simulink library "speedgoatlib_fpga_analog_io"  (R2024b)
settings: Solver=VariableStepAuto  StartTime=0.0  StopTime=10.0  RelTol=1e-3
undefined symbols (not defined in the file): IO336, sg_fpga_callBackInit_m_a1, sg_fpga_io324_analog_input_m, sg_fpga_io324_analog_output_m, sg_fpga_io324_analog_setup_m, sg_fpga_io325_analog_input_m, sg_fpga_io325_analog_output_m, sg_fpga_io325_analog_setup_m, sg_fpga_io334_analog_input_m, sg_fpga_io334_analog_output_m, sg_fpga_io334_analog_setup_m, sg_fpga_io336_analog_input_m, sg_fpga_io336_analog_output_m, sg_fpga_io336_analog_setup_m, sg_fpga_io337_analog_input_m, sg_fpga_io337_analog_output_m, sg_fpga_io337_analog_setup_m, sg_fpga_io3xx_120_analog_input_m, sg_fpga_io3xx_120_analog_output_m, sg_fpga_io3xx_120_analog_setup_m
(part 1 of 4)
settings Model: Creator=Speedgoat GmbH  LastModifiedBy=speedgoat\jenkins
settings DebuggingCC: UnderspecifiedInitializationDetection=Classic  MergeDetectMultiDrivingBlocksExec=none
settings ModelReferenceCC: PropagateSignalLabelsOutOfModel=off
settings ConfigComp: CovBoundaryAbsTol=1.0e-5

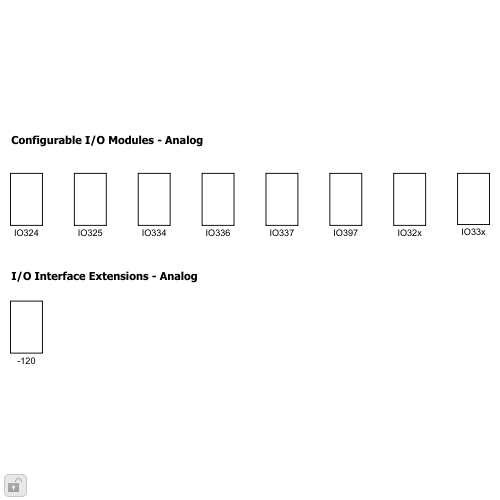
[thumbnail: Simulink's stored preview of the top-level diagram]
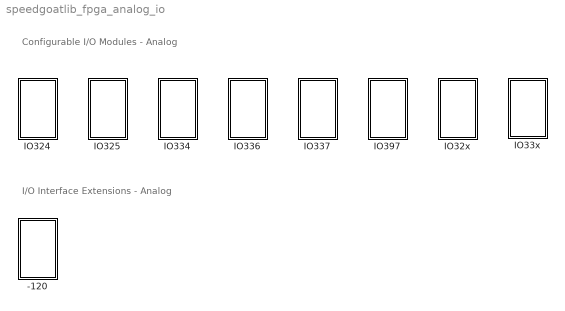
== system speedgoatlib_fpga_analog_io ==
  note: Configurable I/O Modules - Analog
  note: I/O Interface Extensions - Analog
  -120 : Subsystem
  IO324 : Subsystem
  IO325 : Subsystem
  IO32x : Subsystem
  IO334 : Subsystem
  IO336 : Subsystem
  IO337 : Subsystem
  IO33x : Subsystem
  IO397 : Subsystem

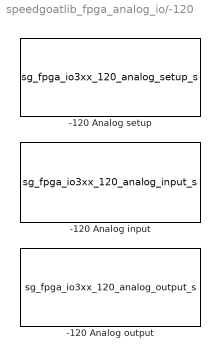
== system speedgoatlib_fpga_analog_io/-120 ==
  -120 Analog input : S-Function  InitFcn=sg_fpga_io3xx_120_analog_input_m.runInitFcn();  FunctionName=sg_fpga_io3xx_120_analog_input_s  Parameters=id, parSampleTime, parAiChannels, parAiChannelsStreamed, parAiEnableFrame, parAiFrameSize  SFunctionDeploymentMode=off  EnableBusSupport=off  mask(ad_fpga_io3xx_120){id=1, parSampleTime=-1, pciSlot=[-1,-1], parAiChannels=[1 2], parAiChannelsStreamed=[1 2], parAiTriggerMode=[2 2], parAiReadPrevValue=0, parAiEnableFrame=0, parAdcCoupling=[1 1 1 1], parAdcContSampling=0, parAdcDmaEnable=0, parAdcActiveDmaDevices=[1 1 1 1], parAiFrameSize=100}
      mask prompts: id "Configurable I/O Module ID"; parSampleTime "Sample Time [s]"
      mask help: Speedgoat Driver Block<br>Configurable I/O - 120 Analog Input<br><br>&copy; 2007 - 2026, Speedgoat GmbH, <a href="matlab: web('www.speedgoat.com','-browser');">www.speedgoat.com</a>
      mask init:
      | sg_fpga_io3xx_120_analog_input_m.runMaskInit();
      mask Help: eval('sg.utils.help.show(''io_main/refentry_120_analog_input_v1'');')
      mask TypeOptions id: 1 | 2 | 3 | 4 | 5 | 6 | 7 | 8 | 9 | 10
      mask Display: disp('Speedgoat\nConfigurable I/O\n-120 Analog input v1\nModule ID: 1');port_label('output',1,'1');port_label('output',2,'2');
  -120 Analog output : S-Function  InitFcn=sg_fpga_io3xx_120_analog_output_m.runInitFcn();  FunctionName=sg_fpga_io3xx_120_analog_output_s  Parameters=id, parSampleTime, parAoChannels, parAoEnableFrame, parAoFrameSize  SFunctionDeploymentMode=off  EnableBusSupport=off  mask(da_fpga_io3xx_120){id=1, parSampleTime=-1, pciSlot=[-1,-1], board=IO336-325k, parAoChannels=[1 2], parAoVoltageRange=[1 1], parDacOverRange=[0 0 0 0 0 0 0 0], parAoInitValues=[0 0], parAoReset=[1 1], parDacSyncOut=1, parAoEnableFrame=0, parDacActiveDmaDevices=[1 1 1 1], parDacDmaLatency=2, parAoFrameSize=1000}
      mask prompts: id "Configurable I/O Module ID"; parSampleTime "Sample Time [s]"
      mask help: Speedgoat Driver Block<br>Configurable I/O - 120 Analog Output<br><br>&copy; 2007 - 2026, Speedgoat GmbH, <a href="matlab: web('www.speedgoat.com','-browser');">www.speedgoat.com</a>
      mask init:
      | sg_fpga_io3xx_120_analog_output_m.runMaskInit();
      mask Help: eval('sg.utils.help.show(''io_main/refentry_120_analog_output_v1'');')
      mask TypeOptions id: 1 | 2 | 3 | 4 | 5 | 6 | 7 | 8 | 9 | 10
      mask Display: disp('Speedgoat\nConfigurable I/O\n-120 Analog output v1\nModule ID: 1');port_label('input',1,'1');port_label('input',2,'2');
  -120 Analog setup : S-Function  InitFcn=sg_fpga_io3xx_120_analog_setup_m.runInitFcn();  FunctionName=sg_fpga_io3xx_120_analog_setup_s  Parameters=id, p.cmcEnable, p.AdcActiveChannels, p.AdcReadPrevValue, p.AdcFilterWidthPow2, p.AdcOversamplRate, parAdcAutoCorrection, p.AdcTriggerMode, p.AdcClockDivider, p.AdcInternalTrigger, p.AdcExternalTrigger, p.AdcEnableFrame, p.AdcFrameSize, p.DacChannels, p.DacVoltageRange, p.DacInitValues, p.DacReset, parDacAutoCorrection, p.DacTriggerMode, p.DacClockDivider, p.DacInternalTrigger, p.DacExternalTrigger, p.DacEnableFrame, p.DacFifoThreshold, p.DacSourceSelection, p.DacFrameSize, p.EnableTriggerForCm, p.DacUsesTimer  SFunctionModules=sg_fpga_analog_dma sg_AnalogInputCm_IO336 sg_AnalogOutputCm_IO334  SFunctionDeploymentMode=off  EnableBusSupport=off  mask(analog_setup_fpga_io3xx_120){id=1, siteIdx=1, parEnableCodeModule1=off, parEnableCodeModule2=off, parEnableCodeModule3=off, parEnableCodeModule4=off, parEnableCodeModule5=off, parEnableCodeModule6=off, parEnableCodeModule7=off, parEnableCodeModule8=off, parAdcEnableIndividualTrigger=off, parAdcTriggerMode1=Model Step, parAdcSampleRate1=1e5, parAdcDioTriggerChannel1=1, parAdcInternalTrigger1=<empty>, parAdcOversampling1=None, parAdcTriggerMode2=Model Step, parAdcSampleRate2=1e5, parAdcDioTriggerChannel2=1, parAdcInternalTrigger2=<empty>, parAdcOversampling2=None, parAdcTriggerMode3=Model Step, parAdcSampleRate3=1e5, parAdcDioTriggerChannel3=1, parAdcInternalTrigger3=<empty>, parAdcOversampling3=None, parAdcTriggerMode4=Model Step, parAdcSampleRate4=1e5, parAdcDioTriggerChannel4=1, parAdcInternalTrigger4=<empty>, parAdcOversampling4=None, parAdcReadPrevValueIndividualTrigger=off, parAdcEnableFrame=off, parAdcTriggerMode=I/O Module Clock, parAdcReadPrevValue=on, parAdcSampleRate=100e3, parAdcDioTriggerChannel=1, parAdcInternalTrigger=<empty>, parAdcOversampling=None, parAdcTriggerResolution=1e-08, parAdcSampleRateFrame=1e5, parAdcFrameSize=100, parAdcSampleTime=-1, parDacTriggerMode=Model Step, parDacInternalTrigger=<empty>, parDacDioTriggerChannel=1, parDacEnableFrame=on, dacUsesTimer=off, parDacFifoThreshold=100, parDacTriggerResolution=1e-08, parDacSampleRate=1e6, parDacFrameSize=1000, parDacSampleTime=-1, parAdcChannel1=on, parAdcChannel2=on, parAdcChannel3=off, parAdcChannel4=off, parAdcChannel5=off, parAdcChannel6=off, parAdcChannel7=off, parAdcChannel8=off, parAdcChannel9=off, parAdcChannel10=off, parAdcChannel11=off, parAdcChannel12=off, parAdcChannel13=off, parAdcChannel14=off, parAdcChannel15=off, parAdcChannel16=off, parAdcChannel17=off, parAdcChannel18=off, parAdcChannel19=off, parAdcChannel20=off, parAdcChannel21=off, parAdcChannel22=off, parAdcChannel23=off, parAdcChannel24=off, parAdcChannel25=off, parAdcChannel26=off, parAdcChannel27=off, parAdcChannel28=off, parAdcChannel29=off, parAdcChannel30=off, parAdcChannel31=off, parAdcChannel32=off, parAdcAutoCorrection=on, parDacChannel1=on, parDacChannel2=on, parDacChannel3=off, parDacChannel4=off, parDacChannel5=off, parDacChannel6=off, parDacChannel7=off, parDacChannel8=off, parDacChannel9=off, parDacChannel10=off, parDacChannel11=off, parDacChannel12=off, parDacChannel13=off, parDacChannel14=off, parDacChannel15=off, parDacChannel16=off, parDacRange1=+-10 V, parDacInitValue1=0, parDacReset1=on, parDacInitValue2=0, parDacReset2=on, parDacRange2=+-10 V, parDacInitValue3=0, parDacReset3=on, parDacRange3=+-10 V, parDacInitValue4=0, parDacReset4=on, parDacRange4=+-10 V, parDacInitValue5=0, parDacReset5=on, parDacRange5=+-10 V, parDacInitValue6=0, parDacReset6=on, parDacRange6=+-10 V, parDacInitValue7=0, parDacReset7=on, parDacRange7=+-10 V, parDacInitValue8=0, parDacReset8=on, parDacRange8=+-10 V, parDacInitValue9=0, parDacReset9=on, parDacRange9=+-10 V, parDacInitValue10=0, parDacReset10=on, parDacRange10=+-10 V, parDacInitValue11=0, parDacReset11=on, parDacRange11=+-10 V, parDacInitValue12=0, parDacReset12=on, parDacRange12=+-10 V, parDacInitValue13=0, parDacReset13=on, parDacRange13=+-10 V, parDacInitValue14=0, parDacReset14=on, parDacRange14=+-10 V, parDacInitValue15=0, parDacReset15=on, parDacRange15=+-10 V, parDacInitValue16=0, parDacReset16=on, parDacRange16=+-10 V, parDacAutoCorrection=on, parDacChannel17=on, parDacChannel18=on, parDacChannel19=off, parDacChannel20=off, parDacChannel21=off, parDacChannel22=off, parDacChannel23=off, parDacChannel24=off, parDacChannel25=off, parDacChannel26=off, parDacChannel27=off, parDacChannel28=off, parDacChannel29=off, parDacChannel30=off, parDacChannel31=off, parDacChannel32=off, parDacRange17=+-10 V, parDacInitValue17=0, parDacReset17=on, parDacInitValue18=0, parDacReset18=on, parDacRange18=+-10 V, parDacInitValue19=0, parDacReset19=on, parDacRange19=+-10 V, parDacInitValue20=0, parDacReset20=on, parDacRange20=+-10 V, parDacInitValue21=0, parDacReset21=on, parDacRange21=+-10 V, parDacInitValue22=0, parDacReset22=on, parDacRange22=+-10 V, parDacInitValue23=0, parDacReset23=on, parDacRange23=+-10 V, parDacInitValue24=0, parDacReset24=on, parDacRange24=+-10 V, parDacInitValue25=0, parDacReset25=on, parDacRange25=+-10 V, parDacInitValue26=0, parDacReset26=on, parDacRange26=+-10 V, parDacInitValue27=0, parDacReset27=on, parDacRange27=+-10 V, parDacInitValue28=0, parDacReset28=on, parDacRange28=+-10 V, parDacInitValue29=0, parDacReset29=on, parDacRange29=+-10 V, parDacInitValue30=0, parDacReset30=on, parDacRange30=+-10 V, parDacInitValue31=0, parDacReset31=on, parDacRange31=+-10 V, parDacInitValue32=0, parDacReset32=on, parDacRange32=+-10 V}
      mask prompts: id "Configurable I/O Module ID"; siteIdx "Site Idx"; parAdcEnableIndividualTrigger "Enable Individual Trigger Settings"; parAdcTriggerMode1 "ADC Sample Trigger"; parAdcSampleRate1 "ADC Sample Rate [Hz]"; parAdcDioTriggerChannel1 "Digital I/O Channel"; parAdcInternalTrigger1 "Internal Signal"; parAdcOversampling1 "Oversampling Factor"; parAdcTriggerMode2 "ADC Sample Trigger"; parAdcSampleRate2 "ADC Sample Rate [Hz]"; parAdcDioTriggerChannel2 "Digital I/O Channel"; parAdcInternalTrigger2 "Internal Signal"; parAdcOversampling2 "Oversampling Factor"; parAdcTriggerMode3 "ADC Sample Trigger"; parAdcSampleRate3 "ADC Sample Rate [Hz]"; parAdcDioTriggerChannel3 "Digital I/O Channel"; parAdcInternalTrigger3 "Internal Signal"; parAdcOversampling3 "Oversampling Factor"; parAdcTriggerMode4 "ADC Sample Trigger"; parAdcSampleRate4 "ADC Sample Rate [Hz]"; parAdcDioTriggerChannel4 "Digital I/O Channel"; parAdcInternalTrigger4 "Internal Signal"; parAdcOversampling4 "Oversampling Factor"; parAdcReadPrevValueIndividualTrigger "Read Value From Previous Model Step"; parAdcEnableFrame "Enable DMA Interrupt"; parAdcTriggerMode "ADC Sample Trigger"; parAdcReadPrevValue "Read Value From Previous Model Step"; parAdcSampleRate "ADC Sample Rate [Hz]"; parAdcDioTriggerChannel "Digital I/O Channel"; parAdcInternalTrigger "Internal Signal"; parAdcOversampling "Oversampling Factor"; parAdcTriggerResolution "Trigger Resolution [s]"; parAdcSampleRateFrame "ADC Sample Rate [Hz]"; parAdcFrameSize "Frame Size (samples/channel)"; parAdcSampleTime "Input Block Sample Time [s]"; parDacTriggerMode "DAC Sample Trigger"; parDacInternalTrigger "Internal Signal"; parDacDioTriggerChannel "Digital I/O Channel"; parDacEnableFrame "Enable DMA Interrupt"; dacUsesTimer "Set Sampling Frequency"; parDacFifoThreshold "FIFO Threshold (samples/channel)"; parDacTriggerResolution "Trigger Resolution [s]"; parDacSampleRate "DAC Sample Rate [Hz]"; parDacFrameSize "Frame Size (samples/channel)"; parDacSampleTime "Output Block Sample Time [s]"; parAdcChannel1 "Ch 01"; parAdcChannel2 "Ch 02"; parAdcChannel3 "Ch 03"; parAdcChannel4 "Ch 04"; parAdcChannel5 "Ch 05"; parAdcChannel6 "Ch 06"; parAdcChannel7 "Ch 07"; parAdcChannel8 "Ch 08"; parAdcChannel9 "Ch 09"; parAdcChannel10 "Ch 10"; parAdcChannel11 "Ch 11"; parAdcChannel12 "Ch 12"; parAdcChannel13 "Ch 13"; parAdcChannel14 "Ch 14"; parAdcChannel15 "Ch 15"; parAdcChannel16 "Ch 16"; parAdcChannel17 "Ch 17"; parAdcChannel18 "Ch 18"; parAdcChannel19 "Ch 19"; parAdcChannel20 "Ch 20"; parAdcChannel21 "Ch 21"; parAdcChannel22 "Ch 22"; parAdcChannel23 "Ch 23"; parAdcChannel24 "Ch 24"; parAdcChannel25 "Ch 25"; parAdcChannel26 "Ch 26"; parAdcChannel27 "Ch 27"; parAdcChannel28 "Ch 28"; parAdcChannel29 "Ch 29"; parAdcChannel30 "Ch 30"; parAdcChannel31 "Ch 31"; parAdcChannel32 "Ch 32"; parAdcAutoCorrection "Automatic Data Correction (for Debugging)"; parDacChannel1 "Ch 1"; parDacChannel2 "Ch 2"; parDacChannel3 "Ch 3"; parDacChannel4 "Ch 4"; parDacChannel5 "Ch 5"; parDacChannel6 "Ch 6"; parDacChannel7 "Ch 7"; parDacChannel8 "Ch 8"; parDacChannel9 "Ch 9"; parDacChannel10 "Ch 10"; parDacChannel11 "Ch 11"; parDacChannel12 "Ch 12"; parDacChannel13 "Ch 13"; parDacChannel14 "Ch 14"; parDacChannel15 "Ch 15"; parDacChannel16 "Ch 16"; parDacRange1 "Output Range"; parDacInitValue1 "Initial Value [V]"; parDacReset1 "Reset to Initial Value"; parDacInitValue2 "Initial Value [V]"; parDacReset2 "Reset to Initial Value"; parDacRange2 "Output Range"; parDacInitValue3 "Initial Value [V]"; parDacReset3 "Reset to Initial Value"; parDacRange3 "Output Range"; parDacInitValue4 "Initial Value [V]"; parDacReset4 "Reset to Initial Value"; parDacRange4 "Output Range"; parDacInitValue5 "Initial Value [V]"; parDacReset5 "Reset to Initial Value"; parDacRange5 "Output Range"; parDacInitValue6 "Initial Value [V]"; parDacReset6 "Reset to Initial Value"; parDacRange6 "Output Range"; parDacInitValue7 "Initial Value [V]"; parDacReset7 "Reset to Initial Value"; parDacRange7 "Output Range"; parDacInitValue8 "Initial Value [V]"; parDacReset8 "Reset to Initial Value"; parDacRange8 "Output Range"; parDacInitValue9 "Initial Value [V]"; parDacReset9 "Reset to Initial Value"; parDacRange9 "Output Range"; parDacInitValue10 "Initial Value [V]"; parDacReset10 "Reset to Initial Value"; parDacRange10 "Output Range"; parDacInitValue11 "Initial Value [V]"; parDacReset11 "Reset to Initial Value"; parDacRange11 "Output Range"; parDacInitValue12 "Initial Value [V]"; parDacReset12 "Reset to Initial Value"; parDacRange12 "Output Range"; parDacInitValue13 "Initial Value [V]"; parDacReset13 "Reset to Initial Value"; parDacRange13 "Output Range"; parDacInitValue14 "Initial Value [V]"; parDacReset14 "Reset to Initial Value"; parDacRange14 "Output Range"; parDacInitValue15 "Initial Value [V]"; parDacReset15 "Reset to Initial Value"; parDacRange15 "Output Range"; parDacInitValue16 "Initial Value [V]"; parDacReset16 "Reset to Initial Value"; parDacRange16 "Output Range"; parDacAutoCorrection "Automatic Data Correction (for Debugging)"; parDacChannel17 "Ch 17"; parDacChannel18 "Ch 18"; parDacChannel19 "Ch 19"; parDacChannel20 "Ch 20"; parDacChannel21 "Ch 21"; parDacChannel22 "Ch 22"; parDacChannel23 "Ch 23"; parDacChannel24 "Ch 24"; parDacChannel25 "Ch 25"; parDacChannel26 "Ch 26"; parDacChannel27 "Ch 27"; parDacChannel28 "Ch 28"; parDacChannel29 "Ch 29"; parDacChannel30 "Ch 30"; parDacChannel31 "Ch 31"; parDacChannel32 "Ch 32"; parDacRange17 "Output Range"; parDacInitValue17 "Initial Value [V]"; parDacReset17 "Reset to Initial Value"; parDacInitValue18 "Initial Value [V]"; parDacReset18 "Reset to Initial Value"; parDacRange18 "Output Range"; parDacInitValue19 "Initial Value [V]"; parDacReset19 "Reset to Initial Value"; parDacRange19 "Output Range"; parDacInitValue20 "Initial Value [V]"; parDacReset20 "Reset to Initial Value"; parDacRange20 "Output Range"; parDacInitValue21 "Initial Value [V]"; parDacReset21 "Reset to Initial Value"; parDacRange21 "Output Range"; parDacInitValue22 "Initial Value [V]"; parDacReset22 "Reset to Initial Value"; parDacRange22 "Output Range"; parDacInitValue23 "Initial Value [V]"; parDacReset23 "Reset to Initial Value"; parDacRange23 "Output Range"; parDacInitValue24 "Initial Value [V]"; parDacReset24 "Reset to Initial Value"; parDacRange24 "Output Range"; parDacInitValue25 "Initial Value [V]"; parDacReset25 "Reset to Initial Value"; parDacRange25 "Output Range"; parDacInitValue26 "Initial Value [V]"; parDacReset26 "Reset to Initial Value"; parDacRange26 "Output Range"; parDacInitValue27 "Initial Value [V]"; parDacReset27 "Reset to Initial Value"; parDacRange27 "Output Range"; parDacInitValue28 "Initial Value [V]"; parDacReset28 "Reset to Initial Value"; parDacRange28 "Output Range"; parDacInitValue29 "Initial Value [V]"; parDacReset29 "Reset to Initial Value"; parDacRange29 "Output Range"; parDacInitValue30 "Initial Value [V]"; parDacReset30 "Reset to Initial Value"; parDacRange30 "Output Range"; parDacInitValue31 "Initial Value [V]"; parDacReset31 "Reset to Initial Value"; parDacRange31 "Output Range"; parDacInitValue32 "Initial Value [V]"; parDacReset32 "Reset to Initial Value"; parDacRange32 "Output Range"
      mask help: Speedgoat Driver Block<br>Configurable I/O - 120 Analog setup<br><br>&copy; 2007 - 2026, Speedgoat GmbH, <a href="matlab: web('www.speedgoat.com','-browser');">www.speedgoat.com</a>
      mask init:
      | p = sg_fpga_io3xx_120_analog_setup_m.runMaskInit();
      settings: OpenFcn=sg_fpga_io3xx_120_analog_setup_m.runOpenMaskCb();
      mask Help: eval('sg.utils.help.show(''io_main/refentry_120_analog_setup_v1'');')
      mask TypeOptions id: 1 | 2 | 3 | 4 | 5 | 6 | 7 | 8 | 9 | 10
      mask TypeOptions siteIdx: 1 | 2
      mask Callback parEnableCodeModule1: sg_fpga_io3xx_120_analog_setup_m.runEnableCmCb(1);
      mask Callback parEnableCodeModule2: sg_fpga_io3xx_120_analog_setup_m.runEnableCmCb(2);
      mask Callback parEnableCodeModule3: sg_fpga_io3xx_120_analog_setup_m.runEnableCmCb(3);
      mask Callback parEnableCodeModule4: sg_fpga_io3xx_120_analog_setup_m.runEnableCmCb(4);
      mask Callback parEnableCodeModule5: sg_fpga_io3xx_120_analog_setup_m.runEnableCmCb(5);
      mask Callback parEnableCodeModule6: sg_fpga_io3xx_120_analog_setup_m.runEnableCmCb(6);
      mask Callback parEnableCodeModule7: sg_fpga_io3xx_120_analog_setup_m.runEnableCmCb(7);
      mask Callback parEnableCodeModule8: sg_fpga_io3xx_120_analog_setup_m.runEnableCmCb(8);
      mask Callback parAdcEnableIndividualTrigger: sg_fpga_io3xx_120_analog_setup_m.runAnalogInputCb();
      mask TypeOptions parAdcTriggerMode1: Model Step | I/O Module Clock | I/O Module Internal Signal | I/O Module Digital I/O
      mask Callback parAdcTriggerMode1: sg_fpga_io3xx_120_analog_setup_m.runAdcTriggerCb('suffix', '1');
      mask TypeOptions parAdcInternalTrigger1: <empty>
      mask TypeOptions parAdcOversampling1: None | 2 | 4 | 8 | 16 | 32 | 64
      mask TypeOptions parAdcTriggerMode2: Model Step | I/O Module Clock | I/O Module Internal Signal | I/O Module Digital I/O
      mask Callback parAdcTriggerMode2: sg_fpga_io3xx_120_analog_setup_m.runAdcTriggerCb('suffix', '2');
      mask TypeOptions parAdcInternalTrigger2: <empty>
      mask TypeOptions parAdcOversampling2: None | 2 | 4 | 8 | 16 | 32 | 64
      mask TypeOptions parAdcTriggerMode3: Model Step | I/O Module Clock | I/O Module Internal Signal | I/O Module Digital I/O
      mask Callback parAdcTriggerMode3: sg_fpga_io3xx_120_analog_setup_m.runAdcTriggerCb('suffix', '3');
      mask TypeOptions parAdcInternalTrigger3: <empty>
      mask TypeOptions parAdcOversampling3: None | 2 | 4 | 8 | 16 | 32 | 64
      mask TypeOptions parAdcTriggerMode4: Model Step | I/O Module Clock | I/O Module Internal Signal | I/O Module Digital I/O
      mask Callback parAdcTriggerMode4: sg_fpga_io3xx_120_analog_setup_m.runAdcTriggerCb('suffix', '4');
      mask TypeOptions parAdcInternalTrigger4: <empty>
      mask TypeOptions parAdcOversampling4: None | 2 | 4 | 8 | 16 | 32 | 64
      mask Callback parAdcEnableFrame: sg_fpga_io3xx_120_analog_setup_m.runEnableFrameCb();
      mask TypeOptions parAdcTriggerMode: Model Step | I/O Module Clock | I/O Module Internal Signal | I/O Module Digital I/O
      mask Callback parAdcTriggerMode: sg_fpga_io3xx_120_analog_setup_m.runAdcTriggerCb();
      mask TypeOptions parAdcInternalTrigger: <empty>
      mask TypeOptions parAdcOversampling: None | 2 | 4 | 8 | 16 | 32 | 64
      mask TypeOptions parDacTriggerMode: Model Step | I/O Module Clock | I/O Module Internal Signal | I/O Module Digital I/O
      mask Callback parDacTriggerMode: sg_fpga_io3xx_120_analog_setup_m.runDacTriggerCb();
      mask TypeOptions parDacInternalTrigger: <empty>
      mask Callback parDacEnableFrame: sg_fpga_io3xx_120_analog_setup_m.runDacTriggerCb();
      mask Callback dacUsesTimer: sg_fpga_io3xx_120_analog_setup_m.runDacTriggerCb();
      mask Callback parAdcChannel1: sg_fpga_io3xx_120_analog_setup_m.runAnalogInputCb();
      mask Callback parAdcChannel2: sg_fpga_io3xx_120_analog_setup_m.runAnalogInputCb();
      mask Callback parAdcChannel3: sg_fpga_io3xx_120_analog_setup_m.runAnalogInputCb();
      mask Callback parAdcChannel4: sg_fpga_io3xx_120_analog_setup_m.runAnalogInputCb();
      mask Callback parAdcChannel5: sg_fpga_io3xx_120_analog_setup_m.runAnalogInputCb();
      mask Callback parAdcChannel6: sg_fpga_io3xx_120_analog_setup_m.runAnalogInputCb();
      mask Callback parAdcChannel7: sg_fpga_io3xx_120_analog_setup_m.runAnalogInputCb();
      mask Callback parAdcChannel8: sg_fpga_io3xx_120_analog_setup_m.runAnalogInputCb();
      mask Callback parAdcChannel9: sg_fpga_io3xx_120_analog_setup_m.runAnalogInputCb();
      mask Callback parAdcChannel10: sg_fpga_io3xx_120_analog_setup_m.runAnalogInputCb();
      mask Callback parAdcChannel11: sg_fpga_io3xx_120_analog_setup_m.runAnalogInputCb();
      mask Callback parAdcChannel12: sg_fpga_io3xx_120_analog_setup_m.runAnalogInputCb();
      mask Callback parAdcChannel13: sg_fpga_io3xx_120_analog_setup_m.runAnalogInputCb();
      mask Callback parAdcChannel14: sg_fpga_io3xx_120_analog_setup_m.runAnalogInputCb();
      mask Callback parAdcChannel15: sg_fpga_io3xx_120_analog_setup_m.runAnalogInputCb();
      mask Callback parAdcChannel16: sg_fpga_io3xx_120_analog_setup_m.runAnalogInputCb();
      mask Callback parAdcChannel17: sg_fpga_io3xx_120_analog_setup_m.runAnalogInputCb();
      mask Callback parAdcChannel18: sg_fpga_io3xx_120_analog_setup_m.runAnalogInputCb();
      mask Callback parAdcChannel19: sg_fpga_io3xx_120_analog_setup_m.runAnalogInputCb();
      mask Callback parAdcChannel20: sg_fpga_io3xx_120_analog_setup_m.runAnalogInputCb();
      mask Callback parAdcChannel21: sg_fpga_io3xx_120_analog_setup_m.runAnalogInputCb();
      mask Callback parAdcChannel22: sg_fpga_io3xx_120_analog_setup_m.runAnalogInputCb();
      mask Callback parAdcChannel23: sg_fpga_io3xx_120_analog_setup_m.runAnalogInputCb();
      mask Callback parAdcChannel24: sg_fpga_io3xx_120_analog_setup_m.runAnalogInputCb();
      mask Callback parAdcChannel25: sg_fpga_io3xx_120_analog_setup_m.runAnalogInputCb();
      mask Callback parAdcChannel26: sg_fpga_io3xx_120_analog_setup_m.runAnalogInputCb();
      mask Callback parAdcChannel27: sg_fpga_io3xx_120_analog_setup_m.runAnalogInputCb();
      mask Callback parAdcChannel28: sg_fpga_io3xx_120_analog_setup_m.runAnalogInputCb();
      mask Callback parAdcChannel29: sg_fpga_io3xx_120_analog_setup_m.runAnalogInputCb();
      mask Callback parAdcChannel30: sg_fpga_io3xx_120_analog_setup_m.runAnalogInputCb();
      mask Callback parAdcChannel31: sg_fpga_io3xx_120_analog_setup_m.runAnalogInputCb();
      mask Callback parAdcChannel32: sg_fpga_io3xx_120_analog_setup_m.runAnalogInputCb();
      mask Callback parDacChannel1: sg_fpga_io3xx_120_analog_setup_m.runAnalogOutputCb();
      mask Callback parDacChannel2: sg_fpga_io3xx_120_analog_setup_m.runAnalogOutputCb();
      mask Callback parDacChannel3: sg_fpga_io3xx_120_analog_setup_m.runAnalogOutputCb();
      mask Callback parDacChannel4: sg_fpga_io3xx_120_analog_setup_m.runAnalogOutputCb();
      mask Callback parDacChannel5: sg_fpga_io3xx_120_analog_setup_m.runAnalogOutputCb();
      mask Callback parDacChannel6: sg_fpga_io3xx_120_analog_setup_m.runAnalogOutputCb();
      mask Callback parDacChannel7: sg_fpga_io3xx_120_analog_setup_m.runAnalogOutputCb();
      mask Callback parDacChannel8: sg_fpga_io3xx_120_analog_setup_m.runAnalogOutputCb();
      mask Callback parDacChannel9: sg_fpga_io3xx_120_analog_setup_m.runAnalogOutputCb();
      mask Callback parDacChannel10: sg_fpga_io3xx_120_analog_setup_m.runAnalogOutputCb();
      mask Callback parDacChannel11: sg_fpga_io3xx_120_analog_setup_m.runAnalogOutputCb();
      mask Callback parDacChannel12: sg_fpga_io3xx_120_analog_setup_m.runAnalogOutputCb();
      mask Callback parDacChannel13: sg_fpga_io3xx_120_analog_setup_m.runAnalogOutputCb();
      mask Callback parDacChannel14: sg_fpga_io3xx_120_analog_setup_m.runAnalogOutputCb();
      mask Callback parDacChannel15: sg_fpga_io3xx_120_analog_setup_m.runAnalogOutputCb();
      mask Callback parDacChannel16: sg_fpga_io3xx_120_analog_setup_m.runAnalogOutputCb();
      mask TypeOptions parDacRange1: +-2.5 V | +-5 V | +-10 V
      mask TypeOptions parDacRange2: +-2.5 V | +-5 V | +-10 V
      mask TypeOptions parDacRange3: +-2.5 V | +-5 V | +-10 V
      mask TypeOptions parDacRange4: +-2.5 V | +-5 V | +-10 V
      mask TypeOptions parDacRange5: +-2.5 V | +-5 V | +-10 V
      mask TypeOptions parDacRange6: +-2.5 V | +-5 V | +-10 V
      mask TypeOptions parDacRange7: +-2.5 V | +-5 V | +-10 V
      mask TypeOptions parDacRange8: +-2.5 V | +-5 V | +-10 V
      mask TypeOptions parDacRange9: +-2.5 V | +-5 V | +-10 V
      mask TypeOptions parDacRange10: +-2.5 V | +-5 V | +-10 V
      mask TypeOptions parDacRange11: +-2.5 V | +-5 V | +-10 V
      mask TypeOptions parDacRange12: +-2.5 V | +-5 V | +-10 V
      mask TypeOptions parDacRange13: +-2.5 V | +-5 V | +-10 V
      mask TypeOptions parDacRange14: +-2.5 V | +-5 V | +-10 V
      mask TypeOptions parDacRange15: +-2.5 V | +-5 V | +-10 V
      mask TypeOptions parDacRange16: +-2.5 V | +-5 V | +-10 V
      mask Callback parDacChannel17: sg_fpga_io3xx_120_analog_setup_m.runAnalogOutputCb();
      mask Callback parDacChannel18: sg_fpga_io3xx_120_analog_setup_m.runAnalogOutputCb();
      mask Callback parDacChannel19: sg_fpga_io3xx_120_analog_setup_m.runAnalogOutputCb();
      mask Callback parDacChannel20: sg_fpga_io3xx_120_analog_setup_m.runAnalogOutputCb();
      mask Callback parDacChannel21: sg_fpga_io3xx_120_analog_setup_m.runAnalogOutputCb();
      mask Callback parDacChannel22: sg_fpga_io3xx_120_analog_setup_m.runAnalogOutputCb();
      mask Callback parDacChannel23: sg_fpga_io3xx_120_analog_setup_m.runAnalogOutputCb();
      mask Callback parDacChannel24: sg_fpga_io3xx_120_analog_setup_m.runAnalogOutputCb();
      mask Callback parDacChannel25: sg_fpga_io3xx_120_analog_setup_m.runAnalogOutputCb();
      mask Callback parDacChannel26: sg_fpga_io3xx_120_analog_setup_m.runAnalogOutputCb();
      mask Callback parDacChannel27: sg_fpga_io3xx_120_analog_setup_m.runAnalogOutputCb();
      mask Callback parDacChannel28: sg_fpga_io3xx_120_analog_setup_m.runAnalogOutputCb();
      mask Callback parDacChannel29: sg_fpga_io3xx_120_analog_setup_m.runAnalogOutputCb();
      mask Callback parDacChannel30: sg_fpga_io3xx_120_analog_setup_m.runAnalogOutputCb();
      mask Callback parDacChannel31: sg_fpga_io3xx_120_analog_setup_m.runAnalogOutputCb();
      mask Callback parDacChannel32: sg_fpga_io3xx_120_analog_setup_m.runAnalogOutputCb();
      mask TypeOptions parDacRange17: +-2.5 V | +-5 V | +-10 V
      mask TypeOptions parDacRange18: +-2.5 V | +-5 V | +-10 V
      mask TypeOptions parDacRange19: +-2.5 V | +-5 V | +-10 V
      mask TypeOptions parDacRange20: +-2.5 V | +-5 V | +-10 V
      mask TypeOptions parDacRange21: +-2.5 V | +-5 V | +-10 V
      mask TypeOptions parDacRange22: +-2.5 V | +-5 V | +-10 V
      mask TypeOptions parDacRange23: +-2.5 V | +-5 V | +-10 V
      mask TypeOptions parDacRange24: +-2.5 V | +-5 V | +-10 V
      mask TypeOptions parDacRange25: +-2.5 V | +-5 V | +-10 V
      mask TypeOptions parDacRange26: +-2.5 V | +-5 V | +-10 V
      mask TypeOptions parDacRange27: +-2.5 V | +-5 V | +-10 V
      mask TypeOptions parDacRange28: +-2.5 V | +-5 V | +-10 V
      mask TypeOptions parDacRange29: +-2.5 V | +-5 V | +-10 V
      mask TypeOptions parDacRange30: +-2.5 V | +-5 V | +-10 V
      mask TypeOptions parDacRange31: +-2.5 V | +-5 V | +-10 V
      mask TypeOptions parDacRange32: +-2.5 V | +-5 V | +-10 V
      mask DialogControl tabMain Prompt: Main
      mask DialogControl boxModuleSettings Prompt: Module Settings
      mask DialogControl boxCodeModules Prompt: Code Module Functionality
      mask DialogControl boxAdcTrigger Prompt: Analog Input Settings
      mask DialogControl boxAdcIndividualTrigger Prompt: Individual Trigger Settings (Sample Based)
      mask DialogControl boxAdcTrigger1 Prompt: Channel 01-08
      mask DialogControl boxAdcTrigger2 Prompt: Channel 09-16
      mask DialogControl boxAdcTrigger3 Prompt: Channel 17-24
      mask DialogControl boxAdcTrigger4 Prompt: Channel 25-32
      mask DialogControl boxAdcCommonTrigger Prompt: Common Trigger Settings
      mask DialogControl boxAdcFrameSettings Prompt: Frame-Based Settings
      mask DialogControl parAdcTriggerResolutionInfo Prompt: placeholder
      mask DialogControl parAdcSampleRateFrameInfo Prompt:
      | => 100 kHz
      | (10 us/sample)
      mask DialogControl parAdcFrameSizeInfo Prompt: => 100
      mask DialogControl parAdcSampleTimeInfo Prompt: => 1 ms
      mask DialogControl boxDacTrigger Prompt: Analog Output Trigger
      mask DialogControl boxDacFrameSettings Prompt: Frame-Based Settings
      mask DialogControl parDacFifoThresholdInfo Prompt: placeholder
      mask DialogControl parDacTriggerResolutionInfo Prompt: placeholder
      mask DialogControl parDacSampleRateInfo Prompt:
      | => 1 MHz
      | (1 us/sample)
      mask DialogControl parDacFrameSizeInfo Prompt: => 1000
      mask DialogControl parDacSampleTimeInfo Prompt: => 1 ms
      mask DialogControl tabAdc Prompt: Analog Inputs
      mask DialogControl tabAdcPosition1 Prompt: Analog Inputs Position 1
      mask DialogControl boxAdc1 Prompt: Channel 01-08
      mask DialogControl boxAdc2 Prompt: Channel 09-16
      mask DialogControl tabAdcPosition2 Prompt: Analog Inputs Position 2
      mask DialogControl boxAdc3 Prompt: Channel 17-24
      mask DialogControl boxAdc4 Prompt: Channel 25-32
      mask DialogControl tabDac Prompt: Analog Outputs
      mask DialogControl tabDacPosition1 Prompt: Analog Outputs Position 1Analog Outputs Position 2
      mask DialogControl boxAoChannels Prompt: Available Channels
      mask DialogControl boxDacRange Prompt: Common Output Voltage Range
      mask DialogControl boxDacSetting Prompt: Channel Settings
      mask DialogControl boxDacChannel1 Prompt: Channel 1
      mask DialogControl boxDacChannel2 Prompt: Channel 2
      mask DialogControl boxDacChannel3 Prompt: Channel 3
      mask DialogControl boxDacChannel4 Prompt: Channel 4
      mask DialogControl boxDacChannel5 Prompt: Channel 5
      mask DialogControl boxDacChannel6 Prompt: Channel 6
      mask DialogControl boxDacChannel7 Prompt: Channel 7
      mask DialogControl boxDacChannel8 Prompt: Channel 8
      mask DialogControl boxDacChannel9 Prompt: Channel 9
      mask DialogControl boxDacChannel10 Prompt: Channel 10
      mask DialogControl boxDacChannel11 Prompt: Channel 11
      mask DialogControl boxDacChannel12 Prompt: Channel 12
      mask DialogControl boxDacChannel13 Prompt: Channel 13
      mask DialogControl boxDacChannel14 Prompt: Channel 14
      mask DialogControl boxDacChannel15 Prompt: Channel 15
      mask DialogControl boxDacChannel16 Prompt: Channel 16
      mask DialogControl tabDacPosition2 Prompt: Analog Outputs Position 2
      mask DialogControl boxAoChannels2 Prompt: Available Channels
      mask DialogControl boxDacRange2 Prompt: Common Output Voltage Range
      mask DialogControl boxDacSetting2 Prompt: Channel Settings
      mask DialogControl boxDacChannel17 Prompt: Channel 17
      mask DialogControl boxDacChannel18 Prompt: Channel 18
      mask DialogControl boxDacChannel19 Prompt: Channel 19
      mask DialogControl boxDacChannel20 Prompt: Channel 20
      mask DialogControl boxDacChannel21 Prompt: Channel 21
      mask DialogControl boxDacChannel22 Prompt: Channel 22
      mask DialogControl boxDacChannel23 Prompt: Channel 23
      mask DialogControl boxDacChannel24 Prompt: Channel 24
      mask DialogControl boxDacChannel25 Prompt: Channel 25
      mask DialogControl boxDacChannel26 Prompt: Channel 26
      mask DialogControl boxDacChannel27 Prompt: Channel 27
      mask DialogControl boxDacChannel28 Prompt: Channel 28
      mask DialogControl boxDacChannel29 Prompt: Channel 29
      mask DialogControl boxDacChannel30 Prompt: Channel 30
      mask DialogControl boxDacChannel31 Prompt: Channel 31
      mask DialogControl boxDacChannel32 Prompt: Channel 32
      mask Display: disp('Speedgoat\nConfigurable I/O\n-120 Analog setup v1\nModule ID: 1');
